simulink model "mobilerobot_DT_SMC"  (R2016b)
settings: Solver=FixedStepAuto  StartTime=0.0  StopTime=20  FixedStep=0.01  RelTol=1e-3
values from neighbouring files (symbols this model uses):
  b = 0.75    [robotprojectvalues.m]
  c = K'    [DTSMC_Gao_TWMR_Position_param.m]    (also in DTSMC_Gao_TWMR_velocity_param.m; robotprojectvalues.m = 0.5)
  c1_pos = c_pos(1)    [robotprojectvalues.m]
  c1_vel = c_vel(1)    [robotprojectvalues.m]
  c2_pos = c_pos(2)    [robotprojectvalues.m]
  c_pos = K_pos'    [robotprojectvalues.m]
  c_vel = K_vel'    [robotprojectvalues.m]
  d = 1    [robotprojectvalues.m]
  dm = 0.1    [robotprojectvalues.m]
  esp = 0.1    [robotprojectvalues.m]
  Gam_tau_pos = [5e-5; 0.01]    [robotprojectvalues.m]
  Gam_tau_vel = [0;1]    [robotprojectvalues.m]
  I_c = 1    [robotprojectvalues.m]
  I_m = 15    [robotprojectvalues.m]
  I_w = 100    [robotprojectvalues.m]
  m1 = a(1)    [robotprojectvalues.m]
  m2 = a(2)    [robotprojectvalues.m]
  m_c = 20    [robotprojectvalues.m]
  m_w = 15    [robotprojectvalues.m]
  mu = 250    [robotprojectvalues.m]
  tau = 0.01    [robotprojectvalues.m]
  x = (1-mu*tau)    (= -1)    [robotprojectvalues.m]
  Xr_c = 5    [robotprojectvalues.m]
  y = dm-esp*tau    (= 0.099)    [robotprojectvalues.m]
  Yr_c = 0    [robotprojectvalues.m]
undefined symbols (not defined in the file or in its folder): fai, Kd, Ki, Kp, theta_dot_L, theta_dot_R
libraries: dspinverses x2, simulink x1
(part 2 of 2)

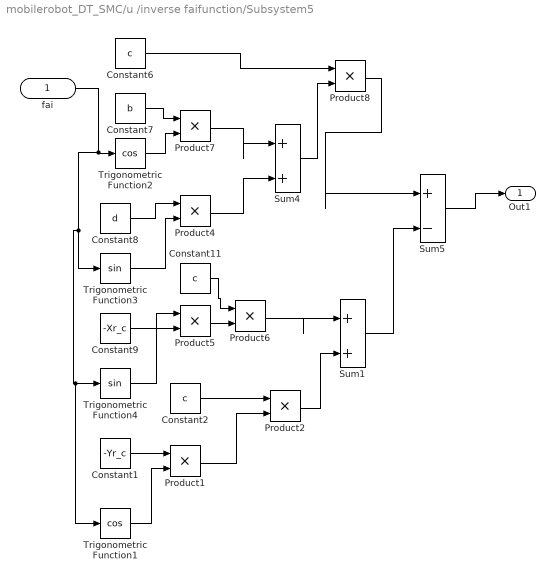
== system mobilerobot_DT_SMC/u /inverse faifunction/Subsystem5 ==
  "fai " : Inport
  Constant1 : Constant  Value=-Yr_c
  Constant11 : Constant  Value=c
  Constant2 : Constant  Value=c
  Constant6 : Constant  Value=c
  Constant7 : Constant  Value=b
  Constant8 : Constant  Value=d
  Constant9 : Constant  Value=-Xr_c
  Product{1..2,4..8} (7 alike) : Product
  Sum1 : Sum  Inputs=|++
  Sum4 : Sum  Inputs=|++
  Sum5 : Sum  Inputs=|+-
  Trigonometric Function1 : Trigonometry  Operator=cos
  Trigonometric Function2 : Trigonometry  Operator=cos
  Trigonometric Function3 : Trigonometry
  Trigonometric Function4 : Trigonometry
  Out1 : Outport
  wires:
  Trigonometric Function3/1 -> Product4/2
  Product7/1 -> Sum4/1
  Trigonometric Function4/1 -> Product5/1
  Constant7/1 -> Product7/1
  Product4/1 -> Sum4/2
  Sum4/1 -> Product8/2
  Constant8/1 -> Product4/1
  Constant9/1 -> Product5/2
  Constant11/1 -> Product6/1
  Product5/1 -> Product6/2
  "fai "/1 -> Trigonometric Function1/1, Trigonometric Function4/1, Trigonometric Function3/1, Trigonometric Function2/1
  Trigonometric Function2/1 -> Product7/2
  Constant6/1 -> Product8/1
  Product8/1 -> Sum5/1
  Sum5/1 -> Out1/1
  Constant1/1 -> Product1/1
  Trigonometric Function1/1 -> Product1/2
  Constant2/1 -> Product2/1
  Product1/1 -> Product2/2
  Product2/1 -> Sum1/2
  Product6/1 -> Sum1/1
  Sum1/1 -> Sum5/2

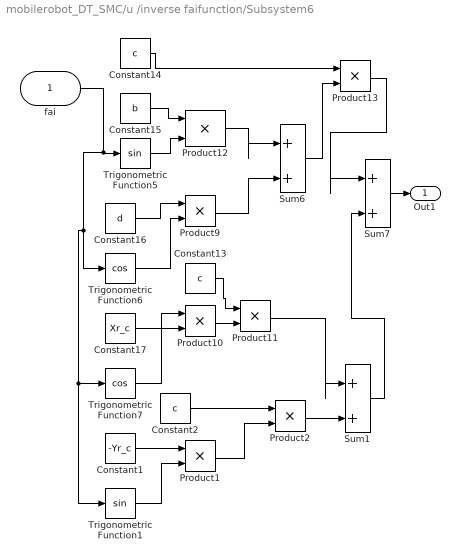
== system mobilerobot_DT_SMC/u /inverse faifunction/Subsystem6 ==
  "fai " : Inport
  Constant1 : Constant  Value=-Yr_c
  Constant13 : Constant  Value=c
  Constant14 : Constant  Value=c
  Constant15 : Constant  Value=b
  Constant16 : Constant  Value=d
  Constant17 : Constant  Value=Xr_c
  Constant2 : Constant  Value=c
  Product{1..2,9..13} (7 alike) : Product
  Sum1 : Sum  Inputs=|++
  Sum6 : Sum  Inputs=|++
  Sum7 : Sum  Inputs=|++
  Trigonometric Function1 : Trigonometry
  Trigonometric Function5 : Trigonometry
  Trigonometric Function6 : Trigonometry  Operator=cos
  Trigonometric Function7 : Trigonometry  Operator=cos
  Out1 : Outport
  wires:
  Sum7/1 -> Out1/1
  Constant16/1 -> Product9/1
  Product9/1 -> Sum6/2
  Product10/1 -> Product11/2
  Constant15/1 -> Product12/1
  Product12/1 -> Sum6/1
  Sum6/1 -> Product13/2
  Trigonometric Function5/1 -> Product12/2
  Product13/1 -> Sum7/1
  Trigonometric Function6/1 -> Product9/2
  Trigonometric Function7/1 -> Product10/1
  Constant14/1 -> Product13/1
  "fai "/1 -> Trigonometric Function1/1, Trigonometric Function7/1, Trigonometric Function6/1, Trigonometric Function5/1
  Constant17/1 -> Product10/2
  Constant13/1 -> Product11/1
  Constant1/1 -> Product1/1
  Trigonometric Function1/1 -> Product1/2
  Constant2/1 -> Product2/1
  Product1/1 -> Product2/2
  Product2/1 -> Sum1/2
  Product11/1 -> Sum1/1
  Sum1/1 -> Sum7/2

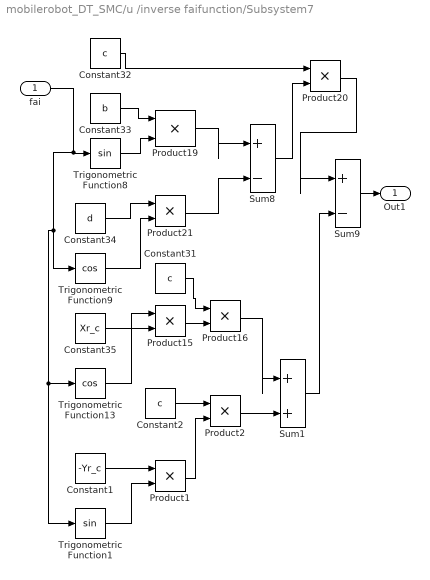
== system mobilerobot_DT_SMC/u /inverse faifunction/Subsystem7 ==
  "fai " : Inport
  Constant1 : Constant  Value=-Yr_c
  Constant2 : Constant  Value=c
  Constant31 : Constant  Value=c
  Constant32 : Constant  Value=c
  Constant33 : Constant  Value=b
  Constant34 : Constant  Value=d
  Constant35 : Constant  Value=Xr_c
  Product{1..2,15..16,19..21} (7 alike) : Product
  Sum1 : Sum  Inputs=|++
  Sum8 : Sum  Inputs=|+-
  Sum9 : Sum  Inputs=|+-
  Trigonometric Function1 : Trigonometry
  Trigonometric Function13 : Trigonometry  Operator=cos
  Trigonometric Function8 : Trigonometry
  Trigonometric Function9 : Trigonometry  Operator=cos
  Out1 : Outport
  wires:
  Product15/1 -> Product16/2
  Constant31/1 -> Product16/1
  Constant34/1 -> Product21/1
  Trigonometric Function8/1 -> Product19/2
  Trigonometric Function13/1 -> Product15/1
  Sum8/1 -> Product20/2
  Constant32/1 -> Product20/1
  Product20/1 -> Sum9/1
  Constant33/1 -> Product19/1
  "fai "/1 -> Trigonometric Function1/1, Trigonometric Function13/1, Trigonometric Function9/1, Trigonometric Function8/1
  Constant35/1 -> Product15/2
  Product21/1 -> Sum8/2
  Product19/1 -> Sum8/1
  Trigonometric Function9/1 -> Product21/2
  Sum9/1 -> Out1/1
  Constant1/1 -> Product1/1
  Trigonometric Function1/1 -> Product1/2
  Constant2/1 -> Product2/1
  Product1/1 -> Product2/2
  Product2/1 -> Sum1/2
  Product16/1 -> Sum1/1
  Sum1/1 -> Sum9/2

== system mobilerobot_DT_SMC/y_2dot=v/Position Model/Subsystem ==
  X1(k-1) : Inport
  X2(k-2) : Inport  Port=2
  Add6 : Sum
  Add7 : Sum  Inputs=+++
  Add9 : Sum  Inputs=+++
  Gain10 : Gain  Gain=-x*c2_pos
  Gain11 : Gain  Gain=y
  Gain12 : Gain  Gain=0.01*c1_pos
  Gain2 : Gain  Gain=c_pos'  Multiplication=Matrix(K*u)
  Gain6 : Gain  Gain=-x*c1_pos
  Gain8 : Gain  Gain=c2_pos
  Gain9 : Gain  Gain=c1_pos
  Matrix Concatenate : Concatenate  Mode=Multidimensional array
  Scope : Scope
  Sign : Signum
  Out1 : Outport
  wires:
  Matrix Concatenate/1 -> Gain2/1
  Gain8/1 -> Add9/2
  Gain10/1 -> Add9/3
  Add9/1 -> Add7/2
  Gain12/1 -> Add9/1
  Gain11/1 -> Add7/3
  Gain6/1 -> Add6/2
  Add6/1 -> Add7/1
  Gain2/1 -> Sign/1  "s(k-1)"
  Gain9/1 -> Add6/1
  Sign/1 -> Scope/1, Gain11/1
  Add7/1 -> Out1/1
  X1(k-1)/1 -> Matrix Concatenate/1, Gain6/1, Gain9/1
  X2(k-2)/1 -> Matrix Concatenate/2, Gain12/1, Gain8/1, Gain10/1

== system mobilerobot_DT_SMC/y_2dot=v/Position Model1/Subsystem ==
  X1(k-1) : Inport
  X2(k-1) : Inport  Port=2
  Add6 : Sum
  Add7 : Sum  Inputs=+++
  Add9 : Sum  Inputs=+++
  Gain10 : Gain  Gain=-x*c2_pos
  Gain11 : Gain  Gain=y
  Gain12 : Gain  Gain=0.01*c1_pos
  Gain2 : Gain  Gain=c_pos'  Multiplication=Matrix(K*u)
  Gain6 : Gain  Gain=-x*c1_pos
  Gain8 : Gain  Gain=c2_pos
  Gain9 : Gain  Gain=c1_pos
  Matrix Concatenate : Concatenate  Mode=Multidimensional array
  Sign : Signum
  Out1 : Outport
  wires:
  Matrix Concatenate/1 -> Gain2/1
  Gain8/1 -> Add9/2
  Gain10/1 -> Add9/3
  Add9/1 -> Add7/2
  Gain12/1 -> Add9/1
  Gain11/1 -> Add7/3
  Gain6/1 -> Add6/2
  Add6/1 -> Add7/1
  Gain2/1 -> Sign/1  "s(k-1)"
  Gain9/1 -> Add6/1
  Sign/1 -> Gain11/1
  Add7/1 -> Out1/1
  X1(k-1)/1 -> Matrix Concatenate/1, Gain6/1, Gain9/1
  X2(k-1)/1 -> Matrix Concatenate/2, Gain12/1, Gain8/1, Gain10/1

== system mobilerobot_DT_SMC/y_2dot=v/Velocity Model/Subsystem1 ==
  X(k-1) : Inport
  u(k-2) : Inport  Port=2
  Add5 : Sum  Inputs=+++
  Gain3 : Gain  Gain=c_vel'  Multiplication=Matrix(K*u)
  Gain6 : Gain  Gain=m1
  Gain7 : Gain  Gain=m2
  Gain8 : Gain  Gain=-(dm-(esp*tau))
  Matrix Concatenate : Concatenate  Mode=Multidimensional array
  Sign : Signum
  Out1 : Outport
  wires:
  Gain7/1 -> Add5/2
  Sign/1 -> Gain8/1
  Gain6/1 -> Add5/1
  Gain8/1 -> Add5/3
  Gain3/1 -> Sign/1  "s(k-1)"
  Add5/1 -> Out1/1
  Matrix Concatenate/1 -> Gain3/1
  X(k-1)/1 -> Gain6/1, Matrix Concatenate/1
  u(k-2)/1 -> Matrix Concatenate/2, Gain7/1

== system mobilerobot_DT_SMC/y_2dot=v/Velocity Model1/Subsystem1 ==
  X(k-1) : Inport
  u(k-2) : Inport  Port=2
  Add5 : Sum  Inputs=+++
  Gain3 : Gain  Gain=c_vel'  Multiplication=Matrix(K*u)
  Gain6 : Gain  Gain=m1
  Gain7 : Gain  Gain=m2
  Gain8 : Gain  Gain=-(dm-(esp*tau))
  Matrix Concatenate : Concatenate  Mode=Multidimensional array
  Sign : Signum
  Out1 : Outport
  wires:
  Gain7/1 -> Add5/2
  Sign/1 -> Gain8/1
  Gain6/1 -> Add5/1
  Gain8/1 -> Add5/3
  Gain3/1 -> Sign/1  "s(k-1)"
  Add5/1 -> Out1/1
  Matrix Concatenate/1 -> Gain3/1
  X(k-1)/1 -> Gain6/1, Matrix Concatenate/1
  u(k-2)/1 -> Matrix Concatenate/2, Gain7/1

== system mobilerobot_DT_SMC/y_2dot=v/xydot/Subsystem4 ==
  "fai " : Inport
  Constant1 : Constant  Value=-Yr_c
  Constant2 : Constant  Value=c
  Constant25 : Constant  Value=c
  Constant26 : Constant  Value=b
  Constant27 : Constant  Value=d
  Constant28 : Constant  Value=-Xr_c
  Constant30 : Constant  Value=c
  Product{1..4,14,17..18} (7 alike) : Product
  Sum1 : Sum  Inputs=|++
  Sum2 : Sum  Inputs=|+-
  Sum3 : Sum  Inputs=|++
  Trigonometric Function1 : Trigonometry  Operator=cos
  Trigonometric Function10 : Trigonometry  Operator=cos
  Trigonometric Function11 : Trigonometry
  Trigonometric Function12 : Trigonometry
  Out1 : Outport
  wires:
  Trigonometric Function10/1 -> Product2/2
  Constant26/1 -> Product2/1
  Product14/1 -> Sum2/2
  Sum2/1 -> Product3/2
  Sum3/1 -> Out1/1
  Trigonometric Function12/1 -> Product17/1
  "fai "/1 -> Trigonometric Function1/1, Trigonometric Function12/1, Trigonometric Function11/1, Trigonometric Function10/1
  Constant27/1 -> Product14/1
  Product17/1 -> Product18/2
  Constant28/1 -> Product17/2
  Trigonometric Function11/1 -> Product14/2
  Constant30/1 -> Product18/1
  Product2/1 -> Sum2/1
  Product3/1 -> Sum3/1
  Constant25/1 -> Product3/1
  Constant1/1 -> Product1/1
  Trigonometric Function1/1 -> Product1/2
  Constant2/1 -> Product4/1
  Product1/1 -> Product4/2
  Product4/1 -> Sum1/2
  Product18/1 -> Sum1/1
  Sum1/1 -> Sum3/2

== system mobilerobot_DT_SMC/y_2dot=v/xydot/Subsystem5 ==
  "fai " : Inport
  Constant1 : Constant  Value=-Yr_c
  Constant11 : Constant  Value=c
  Constant2 : Constant  Value=c
  Constant6 : Constant  Value=c
  Constant7 : Constant  Value=b
  Constant8 : Constant  Value=d
  Constant9 : Constant  Value=-Xr_c
  Product{1..2,4..8} (7 alike) : Product
  Sum1 : Sum  Inputs=|++
  Sum4 : Sum  Inputs=|++
  Sum5 : Sum  Inputs=|+-
  Trigonometric Function1 : Trigonometry  Operator=cos
  Trigonometric Function2 : Trigonometry  Operator=cos
  Trigonometric Function3 : Trigonometry
  Trigonometric Function4 : Trigonometry
  Out1 : Outport
  wires:
  Trigonometric Function3/1 -> Product4/2
  Product7/1 -> Sum4/1
  Trigonometric Function4/1 -> Product5/1
  Constant7/1 -> Product7/1
  Product4/1 -> Sum4/2
  Sum4/1 -> Product8/2
  Constant8/1 -> Product4/1
  Constant9/1 -> Product5/2
  Constant11/1 -> Product6/1
  Product5/1 -> Product6/2
  "fai "/1 -> Trigonometric Function1/1, Trigonometric Function4/1, Trigonometric Function3/1, Trigonometric Function2/1
  Trigonometric Function2/1 -> Product7/2
  Constant6/1 -> Product8/1
  Product8/1 -> Sum5/1
  Sum5/1 -> Out1/1
  Constant1/1 -> Product1/1
  Trigonometric Function1/1 -> Product1/2
  Constant2/1 -> Product2/1
  Product1/1 -> Product2/2
  Product2/1 -> Sum1/2
  Product6/1 -> Sum1/1
  Sum1/1 -> Sum5/2

== system mobilerobot_DT_SMC/y_2dot=v/xydot/Subsystem6 ==
  "fai " : Inport
  Constant1 : Constant  Value=-Yr_c
  Constant13 : Constant  Value=c
  Constant14 : Constant  Value=c
  Constant15 : Constant  Value=b
  Constant16 : Constant  Value=d
  Constant17 : Constant  Value=Xr_c
  Constant2 : Constant  Value=c
  Product{1..2,9..13} (7 alike) : Product
  Sum1 : Sum  Inputs=|++
  Sum6 : Sum  Inputs=|++
  Sum7 : Sum  Inputs=|++
  Trigonometric Function1 : Trigonometry
  Trigonometric Function5 : Trigonometry
  Trigonometric Function6 : Trigonometry  Operator=cos
  Trigonometric Function7 : Trigonometry  Operator=cos
  Out1 : Outport
  wires:
  Sum7/1 -> Out1/1
  Constant16/1 -> Product9/1
  Product9/1 -> Sum6/2
  Product10/1 -> Product11/2
  Constant15/1 -> Product12/1
  Product12/1 -> Sum6/1
  Sum6/1 -> Product13/2
  Trigonometric Function5/1 -> Product12/2
  Product13/1 -> Sum7/1
  Trigonometric Function6/1 -> Product9/2
  Trigonometric Function7/1 -> Product10/1
  Constant14/1 -> Product13/1
  "fai "/1 -> Trigonometric Function1/1, Trigonometric Function7/1, Trigonometric Function6/1, Trigonometric Function5/1
  Constant17/1 -> Product10/2
  Constant13/1 -> Product11/1
  Constant1/1 -> Product1/1
  Trigonometric Function1/1 -> Product1/2
  Constant2/1 -> Product2/1
  Product1/1 -> Product2/2
  Product2/1 -> Sum1/2
  Product11/1 -> Sum1/1
  Sum1/1 -> Sum7/2

== system mobilerobot_DT_SMC/y_2dot=v/xydot/Subsystem7 ==
  "fai " : Inport
  Constant1 : Constant  Value=-Yr_c
  Constant2 : Constant  Value=c
  Constant31 : Constant  Value=c
  Constant32 : Constant  Value=c
  Constant33 : Constant  Value=b
  Constant34 : Constant  Value=d
  Constant35 : Constant  Value=Xr_c
  Product{1..2,15..16,19..21} (7 alike) : Product
  Sum1 : Sum  Inputs=|++
  Sum8 : Sum  Inputs=|+-
  Sum9 : Sum  Inputs=|+-
  Trigonometric Function1 : Trigonometry
  Trigonometric Function13 : Trigonometry  Operator=cos
  Trigonometric Function8 : Trigonometry
  Trigonometric Function9 : Trigonometry  Operator=cos
  Out1 : Outport
  wires:
  Product15/1 -> Product16/2
  Constant31/1 -> Product16/1
  Constant34/1 -> Product21/1
  Trigonometric Function8/1 -> Product19/2
  Trigonometric Function13/1 -> Product15/1
  Sum8/1 -> Product20/2
  Constant32/1 -> Product20/1
  Product20/1 -> Sum9/1
  Constant33/1 -> Product19/1
  "fai "/1 -> Trigonometric Function1/1, Trigonometric Function13/1, Trigonometric Function9/1, Trigonometric Function8/1
  Constant35/1 -> Product15/2
  Product21/1 -> Sum8/2
  Product19/1 -> Sum8/1
  Trigonometric Function9/1 -> Product21/2
  Sum9/1 -> Out1/1
  Constant1/1 -> Product1/1
  Trigonometric Function1/1 -> Product1/2
  Constant2/1 -> Product2/1
  Product1/1 -> Product2/2
  Product2/1 -> Sum1/2
  Product16/1 -> Sum1/1
  Sum1/1 -> Sum9/2

== system mobilerobot_DT_SMC/tau/f2/M/Subsystem ==
  "fai " : Inport
  Constant : Constant  Value=-m_c
  Constant1 : Constant  Value=d
  Product : Product
  Product1 : Product
  Trigonometric Function : Trigonometry
  Out1 : Outport
  wires:
  Trigonometric Function/1 -> Product/2
  "fai "/1 -> Trigonometric Function/1
  Constant/1 -> Product1/1
  Constant1/1 -> Product/1
  Product1/1 -> Out1/1
  Product/1 -> Product1/2

== system mobilerobot_DT_SMC/tau/f2/M/Subsystem1 ==
  fai : Inport
  Constant3 : Constant  Value=m_c
  Constant4 : Constant  Value=d
  Product2 : Product
  Product3 : Product
  Trigonometric Function1 : Trigonometry
  Out1 : Outport
  wires:
  Trigonometric Function1/1 -> Product2/2
  Constant4/1 -> Product2/1
  fai/1 -> Trigonometric Function1/1
  Product2/1 -> Product3/2
  Constant3/1 -> Product3/1
  Product3/1 -> Out1/1

== system mobilerobot_DT_SMC/tau/f2/M1/Subsystem ==
  "fai " : Inport
  Constant : Constant  Value=-m_c
  Constant1 : Constant  Value=d
  Product : Product
  Product1 : Product
  Trigonometric Function : Trigonometry
  Out1 : Outport
  wires:
  Trigonometric Function/1 -> Product/2
  "fai "/1 -> Trigonometric Function/1
  Constant/1 -> Product1/1
  Constant1/1 -> Product/1
  Product1/1 -> Out1/1
  Product/1 -> Product1/2

== system mobilerobot_DT_SMC/tau/f2/M1/Subsystem1 ==
  fai : Inport
  Constant3 : Constant  Value=m_c
  Constant4 : Constant  Value=d
  Product2 : Product
  Product3 : Product
  Trigonometric Function1 : Trigonometry
  Out1 : Outport
  wires:
  Trigonometric Function1/1 -> Product2/2
  Constant4/1 -> Product2/1
  fai/1 -> Trigonometric Function1/1
  Product2/1 -> Product3/2
  Constant3/1 -> Product3/1
  Product3/1 -> Out1/1

== system mobilerobot_DT_SMC/tau/f2/S/Subsystem ==
  "fai " : Inport
  Constant16 : Constant  Value=c
  Constant17 : Constant  Value=b
  Constant18 : Constant
  Product11 : Product
  Product12 : Product
  Product13 : Product
  Sum5 : Sum  Inputs=|+-
  Trigonometric Function8 : Trigonometry
  Trigonometric Function9 : Trigonometry  Operator=cos
  Out1 : Outport
  wires:
  Constant17/1 -> Product13/1
  Product12/1 -> Sum5/2
  Product13/1 -> Sum5/1
  Constant16/1 -> Product11/1
  Product11/1 -> Out1/1
  Constant18/1 -> Product12/1
  Sum5/1 -> Product11/2
  Trigonometric Function8/1 -> Product13/2
  Trigonometric Function9/1 -> Product12/2
  "fai "/1 -> Trigonometric Function9/1, Trigonometric Function8/1

== system mobilerobot_DT_SMC/tau/f2/S/Subsystem1 ==
  "fai " : Inport
  Constant13 : Constant  Value=c
  Constant14 : Constant  Value=b
  Constant15 : Constant
  Product10 : Product
  Product8 : Product
  Product9 : Product
  Sum4 : Sum  Inputs=|++
  Trigonometric Function6 : Trigonometry
  Trigonometric Function7 : Trigonometry  Operator=cos
  Out1 : Outport
  wires:
  Product10/1 -> Out1/1
  Sum4/1 -> Product10/2
  Product9/1 -> Sum4/1
  Trigonometric Function6/1 -> Product9/2
  Product8/1 -> Sum4/2
  Constant14/1 -> Product9/1
  Constant15/1 -> Product8/1
  Trigonometric Function7/1 -> Product8/2
  Constant13/1 -> Product10/1
  "fai "/1 -> Trigonometric Function7/1, Trigonometric Function6/1

== system mobilerobot_DT_SMC/tau/f2/S/Subsystem2 ==
  "fai " : Inport
  Constant10 : Constant  Value=c
  Constant11 : Constant  Value=b
  Constant12 : Constant
  Product5 : Product
  Product6 : Product
  Product7 : Product
  Sum3 : Sum  Inputs=|++
  Trigonometric Function4 : Trigonometry  Operator=cos
  Trigonometric Function5 : Trigonometry
  Out1 : Outport
  wires:
  Constant11/1 -> Product6/1
  Trigonometric Function4/1 -> Product6/2
  Constant12/1 -> Product5/1
  Trigonometric Function5/1 -> Product5/2
  Product6/1 -> Sum3/1
  Product5/1 -> Sum3/2
  Constant10/1 -> Product7/1
  Sum3/1 -> Product7/2
  Product7/1 -> Out1/1
  "fai "/1 -> Trigonometric Function5/1, Trigonometric Function4/1

== system mobilerobot_DT_SMC/tau/f2/S/Subsystem3 ==
  "fai " : Inport
  Constant6 : Constant  Value=c
  Constant7 : Constant  Value=b
  Constant8 : Constant
  Product2 : Product
  Product3 : Product
  Product4 : Product
  Sum2 : Sum  Inputs=|+-
  Trigonometric Function2 : Trigonometry  Operator=cos
  Trigonometric Function3 : Trigonometry
  Out1 : Outport
  wires:
  Sum2/1 -> Product4/2
  Trigonometric Function3/1 -> Product2/2
  Constant8/1 -> Product2/1
  Trigonometric Function2/1 -> Product3/2
  Constant7/1 -> Product3/1
  Product3/1 -> Sum2/1
  Constant6/1 -> Product4/1
  Product2/1 -> Sum2/2
  Product4/1 -> Out1/1
  "fai "/1 -> Trigonometric Function3/1, Trigonometric Function2/1

== system mobilerobot_DT_SMC/tau/f2/S1/Subsystem ==
  "fai " : Inport
  Constant16 : Constant  Value=c
  Constant17 : Constant  Value=b
  Constant18 : Constant
  Product11 : Product
  Product12 : Product
  Product13 : Product
  Sum5 : Sum  Inputs=|+-
  Trigonometric Function8 : Trigonometry
  Trigonometric Function9 : Trigonometry  Operator=cos
  Out1 : Outport
  wires:
  Constant17/1 -> Product13/1
  Product12/1 -> Sum5/2
  Product13/1 -> Sum5/1
  Constant16/1 -> Product11/1
  Product11/1 -> Out1/1
  Constant18/1 -> Product12/1
  Sum5/1 -> Product11/2
  Trigonometric Function8/1 -> Product13/2
  Trigonometric Function9/1 -> Product12/2
  "fai "/1 -> Trigonometric Function9/1, Trigonometric Function8/1

== system mobilerobot_DT_SMC/tau/f2/S1/Subsystem1 ==
  "fai " : Inport
  Constant13 : Constant  Value=c
  Constant14 : Constant  Value=b
  Constant15 : Constant
  Product10 : Product
  Product8 : Product
  Product9 : Product
  Sum4 : Sum  Inputs=|++
  Trigonometric Function6 : Trigonometry
  Trigonometric Function7 : Trigonometry  Operator=cos
  Out1 : Outport
  wires:
  Product10/1 -> Out1/1
  Sum4/1 -> Product10/2
  Product9/1 -> Sum4/1
  Trigonometric Function6/1 -> Product9/2
  Product8/1 -> Sum4/2
  Constant14/1 -> Product9/1
  Constant15/1 -> Product8/1
  Trigonometric Function7/1 -> Product8/2
  Constant13/1 -> Product10/1
  "fai "/1 -> Trigonometric Function7/1, Trigonometric Function6/1

== system mobilerobot_DT_SMC/tau/f2/S1/Subsystem2 ==
  "fai " : Inport
  Constant10 : Constant  Value=c
  Constant11 : Constant  Value=b
  Constant12 : Constant
  Product5 : Product
  Product6 : Product
  Product7 : Product
  Sum3 : Sum  Inputs=|++
  Trigonometric Function4 : Trigonometry  Operator=cos
  Trigonometric Function5 : Trigonometry
  Out1 : Outport
  wires:
  Constant11/1 -> Product6/1
  Trigonometric Function4/1 -> Product6/2
  Constant12/1 -> Product5/1
  Trigonometric Function5/1 -> Product5/2
  Product6/1 -> Sum3/1
  Product5/1 -> Sum3/2
  Constant10/1 -> Product7/1
  Sum3/1 -> Product7/2
  Product7/1 -> Out1/1
  "fai "/1 -> Trigonometric Function5/1, Trigonometric Function4/1

== system mobilerobot_DT_SMC/tau/f2/S1/Subsystem3 ==
  "fai " : Inport
  Constant6 : Constant  Value=c
  Constant7 : Constant  Value=b
  Constant8 : Constant
  Product2 : Product
  Product3 : Product
  Product4 : Product
  Sum2 : Sum  Inputs=|+-
  Trigonometric Function2 : Trigonometry  Operator=cos
  Trigonometric Function3 : Trigonometry
  Out1 : Outport
  wires:
  Sum2/1 -> Product4/2
  Trigonometric Function3/1 -> Product2/2
  Constant8/1 -> Product2/1
  Trigonometric Function2/1 -> Product3/2
  Constant7/1 -> Product3/1
  Product3/1 -> Sum2/1
  Constant6/1 -> Product4/1
  Product2/1 -> Sum2/2
  Product4/1 -> Out1/1
  "fai "/1 -> Trigonometric Function3/1, Trigonometric Function2/1

== system mobilerobot_DT_SMC/tau/f2/S_transpose /Subsystem ==
  "fai " : Inport
  Constant16 : Constant  Value=c
  Constant17 : Constant  Value=b
  Constant18 : Constant
  Product11 : Product
  Product12 : Product
  Product13 : Product
  Sum5 : Sum  Inputs=|+-
  Trigonometric Function8 : Trigonometry
  Trigonometric Function9 : Trigonometry  Operator=cos
  Out1 : Outport
  wires:
  Constant17/1 -> Product13/1
  Product12/1 -> Sum5/2
  Product13/1 -> Sum5/1
  Constant16/1 -> Product11/1
  Product11/1 -> Out1/1
  Constant18/1 -> Product12/1
  Sum5/1 -> Product11/2
  Trigonometric Function8/1 -> Product13/2
  Trigonometric Function9/1 -> Product12/2
  "fai "/1 -> Trigonometric Function9/1, Trigonometric Function8/1

== system mobilerobot_DT_SMC/tau/f2/S_transpose /Subsystem1 ==
  "fai " : Inport
  Constant13 : Constant  Value=c
  Constant14 : Constant  Value=b
  Constant15 : Constant
  Product10 : Product
  Product8 : Product
  Product9 : Product
  Sum4 : Sum  Inputs=|++
  Trigonometric Function6 : Trigonometry
  Trigonometric Function7 : Trigonometry  Operator=cos
  Out1 : Outport
  wires:
  Product10/1 -> Out1/1
  Sum4/1 -> Product10/2
  Product9/1 -> Sum4/1
  Trigonometric Function6/1 -> Product9/2
  Product8/1 -> Sum4/2
  Constant14/1 -> Product9/1
  Constant15/1 -> Product8/1
  Trigonometric Function7/1 -> Product8/2
  Constant13/1 -> Product10/1
  "fai "/1 -> Trigonometric Function7/1, Trigonometric Function6/1

== system mobilerobot_DT_SMC/tau/f2/S_transpose /Subsystem2 ==
  "fai " : Inport
  Constant10 : Constant  Value=c
  Constant11 : Constant  Value=b
  Constant12 : Constant
  Product5 : Product
  Product6 : Product
  Product7 : Product
  Sum3 : Sum  Inputs=|++
  Trigonometric Function4 : Trigonometry  Operator=cos
  Trigonometric Function5 : Trigonometry
  Out1 : Outport
  wires:
  Constant11/1 -> Product6/1
  Trigonometric Function4/1 -> Product6/2
  Constant12/1 -> Product5/1
  Trigonometric Function5/1 -> Product5/2
  Product6/1 -> Sum3/1
  Product5/1 -> Sum3/2
  Constant10/1 -> Product7/1
  Sum3/1 -> Product7/2
  Product7/1 -> Out1/1
  "fai "/1 -> Trigonometric Function5/1, Trigonometric Function4/1

== system mobilerobot_DT_SMC/tau/f2/S_transpose /Subsystem3 ==
  "fai " : Inport
  Constant6 : Constant  Value=c
  Constant7 : Constant  Value=b
  Constant8 : Constant
  Product2 : Product
  Product3 : Product
  Product4 : Product
  Sum2 : Sum  Inputs=|+-
  Trigonometric Function2 : Trigonometry  Operator=cos
  Trigonometric Function3 : Trigonometry
  Out1 : Outport
  wires:
  Sum2/1 -> Product4/2
  Trigonometric Function3/1 -> Product2/2
  Constant8/1 -> Product2/1
  Trigonometric Function2/1 -> Product3/2
  Constant7/1 -> Product3/1
  Product3/1 -> Sum2/1
  Constant6/1 -> Product4/1
  Product2/1 -> Sum2/2
  Product4/1 -> Out1/1
  "fai "/1 -> Trigonometric Function3/1, Trigonometric Function2/1

== system mobilerobot_DT_SMC/tau/f2/S_transpose 1/Subsystem ==
  "fai " : Inport
  Constant16 : Constant  Value=c
  Constant17 : Constant  Value=b
  Constant18 : Constant
  Product11 : Product
  Product12 : Product
  Product13 : Product
  Sum5 : Sum  Inputs=|+-
  Trigonometric Function8 : Trigonometry
  Trigonometric Function9 : Trigonometry  Operator=cos
  Out1 : Outport
  wires:
  Constant17/1 -> Product13/1
  Product12/1 -> Sum5/2
  Product13/1 -> Sum5/1
  Constant16/1 -> Product11/1
  Product11/1 -> Out1/1
  Constant18/1 -> Product12/1
  Sum5/1 -> Product11/2
  Trigonometric Function8/1 -> Product13/2
  Trigonometric Function9/1 -> Product12/2
  "fai "/1 -> Trigonometric Function9/1, Trigonometric Function8/1

== system mobilerobot_DT_SMC/tau/f2/S_transpose 1/Subsystem1 ==
  "fai " : Inport
  Constant13 : Constant  Value=c
  Constant14 : Constant  Value=b
  Constant15 : Constant
  Product10 : Product
  Product8 : Product
  Product9 : Product
  Sum4 : Sum  Inputs=|++
  Trigonometric Function6 : Trigonometry
  Trigonometric Function7 : Trigonometry  Operator=cos
  Out1 : Outport
  wires:
  Product10/1 -> Out1/1
  Sum4/1 -> Product10/2
  Product9/1 -> Sum4/1
  Trigonometric Function6/1 -> Product9/2
  Product8/1 -> Sum4/2
  Constant14/1 -> Product9/1
  Constant15/1 -> Product8/1
  Trigonometric Function7/1 -> Product8/2
  Constant13/1 -> Product10/1
  "fai "/1 -> Trigonometric Function7/1, Trigonometric Function6/1

== system mobilerobot_DT_SMC/tau/f2/S_transpose 1/Subsystem2 ==
  "fai " : Inport
  Constant10 : Constant  Value=c
  Constant11 : Constant  Value=b
  Constant12 : Constant
  Product5 : Product
  Product6 : Product
  Product7 : Product
  Sum3 : Sum  Inputs=|++
  Trigonometric Function4 : Trigonometry  Operator=cos
  Trigonometric Function5 : Trigonometry
  Out1 : Outport
  wires:
  Constant11/1 -> Product6/1
  Trigonometric Function4/1 -> Product6/2
  Constant12/1 -> Product5/1
  Trigonometric Function5/1 -> Product5/2
  Product6/1 -> Sum3/1
  Product5/1 -> Sum3/2
  Constant10/1 -> Product7/1
  Sum3/1 -> Product7/2
  Product7/1 -> Out1/1
  "fai "/1 -> Trigonometric Function5/1, Trigonometric Function4/1

== system mobilerobot_DT_SMC/tau/f2/S_transpose 1/Subsystem3 ==
  "fai " : Inport
  Constant6 : Constant  Value=c
  Constant7 : Constant  Value=b
  Constant8 : Constant
  Product2 : Product
  Product3 : Product
  Product4 : Product
  Sum2 : Sum  Inputs=|+-
  Trigonometric Function2 : Trigonometry  Operator=cos
  Trigonometric Function3 : Trigonometry
  Out1 : Outport
  wires:
  Sum2/1 -> Product4/2
  Trigonometric Function3/1 -> Product2/2
  Constant8/1 -> Product2/1
  Trigonometric Function2/1 -> Product3/2
  Constant7/1 -> Product3/1
  Product3/1 -> Sum2/1
  Constant6/1 -> Product4/1
  Product2/1 -> Sum2/2
  Product4/1 -> Out1/1
  "fai "/1 -> Trigonometric Function3/1, Trigonometric Function2/1

== system mobilerobot_DT_SMC/tau/f2/S_transpose 2/Subsystem ==
  "fai " : Inport
  Constant16 : Constant  Value=c
  Constant17 : Constant  Value=b
  Constant18 : Constant
  Product11 : Product
  Product12 : Product
  Product13 : Product
  Sum5 : Sum  Inputs=|+-
  Trigonometric Function8 : Trigonometry
  Trigonometric Function9 : Trigonometry  Operator=cos
  Out1 : Outport
  wires:
  Constant17/1 -> Product13/1
  Product12/1 -> Sum5/2
  Product13/1 -> Sum5/1
  Constant16/1 -> Product11/1
  Product11/1 -> Out1/1
  Constant18/1 -> Product12/1
  Sum5/1 -> Product11/2
  Trigonometric Function8/1 -> Product13/2
  Trigonometric Function9/1 -> Product12/2
  "fai "/1 -> Trigonometric Function9/1, Trigonometric Function8/1

== system mobilerobot_DT_SMC/tau/f2/S_transpose 2/Subsystem1 ==
  "fai " : Inport
  Constant13 : Constant  Value=c
  Constant14 : Constant  Value=b
  Constant15 : Constant
  Product10 : Product
  Product8 : Product
  Product9 : Product
  Sum4 : Sum  Inputs=|++
  Trigonometric Function6 : Trigonometry
  Trigonometric Function7 : Trigonometry  Operator=cos
  Out1 : Outport
  wires:
  Product10/1 -> Out1/1
  Sum4/1 -> Product10/2
  Product9/1 -> Sum4/1
  Trigonometric Function6/1 -> Product9/2
  Product8/1 -> Sum4/2
  Constant14/1 -> Product9/1
  Constant15/1 -> Product8/1
  Trigonometric Function7/1 -> Product8/2
  Constant13/1 -> Product10/1
  "fai "/1 -> Trigonometric Function7/1, Trigonometric Function6/1

== system mobilerobot_DT_SMC/tau/f2/S_transpose 2/Subsystem2 ==
  "fai " : Inport
  Constant10 : Constant  Value=c
  Constant11 : Constant  Value=b
  Constant12 : Constant
  Product5 : Product
  Product6 : Product
  Product7 : Product
  Sum3 : Sum  Inputs=|++
  Trigonometric Function4 : Trigonometry  Operator=cos
  Trigonometric Function5 : Trigonometry
  Out1 : Outport
  wires:
  Constant11/1 -> Product6/1
  Trigonometric Function4/1 -> Product6/2
  Constant12/1 -> Product5/1
  Trigonometric Function5/1 -> Product5/2
  Product6/1 -> Sum3/1
  Product5/1 -> Sum3/2
  Constant10/1 -> Product7/1
  Sum3/1 -> Product7/2
  Product7/1 -> Out1/1
  "fai "/1 -> Trigonometric Function5/1, Trigonometric Function4/1

== system mobilerobot_DT_SMC/tau/f2/S_transpose 2/Subsystem3 ==
  "fai " : Inport
  Constant6 : Constant  Value=c
  Constant7 : Constant  Value=b
  Constant8 : Constant
  Product2 : Product
  Product3 : Product
  Product4 : Product
  Sum2 : Sum  Inputs=|+-
  Trigonometric Function2 : Trigonometry  Operator=cos
  Trigonometric Function3 : Trigonometry
  Out1 : Outport
  wires:
  Sum2/1 -> Product4/2
  Trigonometric Function3/1 -> Product2/2
  Constant8/1 -> Product2/1
  Trigonometric Function2/1 -> Product3/2
  Constant7/1 -> Product3/1
  Product3/1 -> Sum2/1
  Constant6/1 -> Product4/1
  Product2/1 -> Sum2/2
  Product4/1 -> Out1/1
  "fai "/1 -> Trigonometric Function3/1, Trigonometric Function2/1
